simulink model "SingePhase_FB_Inverter_SPWM"  (R2023a)
settings: Solver=ode23t  StartTime=0.0  StopTime=0.1  MaxStep=1e-4  RelTol=1e-3
libraries: spsMosfetLib x8, spsSeriesRLCBranchLib x6, simulink x3, spsDCVoltageSourceLib x2, spsVoltageMeasurementLib x2, sps_lib x1
settings Model: Creator=Alielden  LastModifiedBy=Alielden
settings DataIOCC: SaveState=on  SignalLogging=off  DSMLogging=off  ReturnWorkspaceOutputs=off  LoggingToFile=on

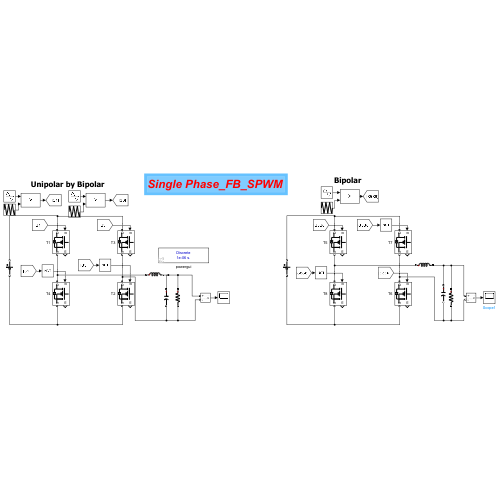
[thumbnail: Simulink's stored preview of the top-level diagram]
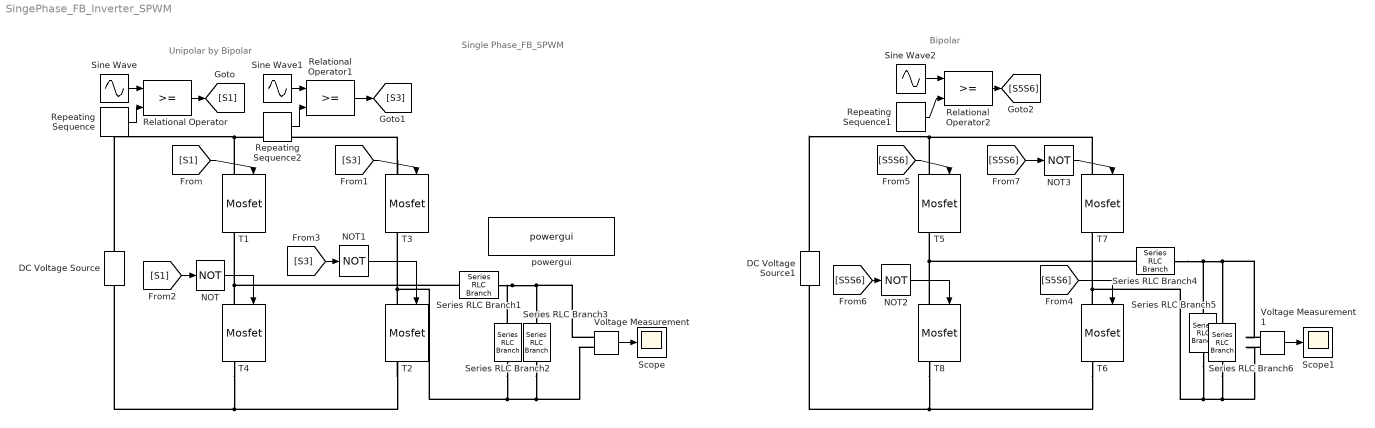
== system SingePhase_FB_Inverter_SPWM ==
  note: Unipolar by Bipolar
  note: Bipolar
  note: Single Phase_FB_SPWM
  DC Voltage Source : spsDCVoltageSourceLib/DC Voltage Source  Amplitude=100  Measurements=None
  DC Voltage Source1 : spsDCVoltageSourceLib/DC Voltage Source  Amplitude=100  Measurements=None
  NOT{,1..3} (4 alike) : Logic  Operator=NOT  AllPortsSameDT=off  OutDataTypeStr=boolean
  Relational Operator : RelationalOperator  OutDataTypeStr=boolean  RndMeth=Simplest  InputSameDT=off
  Relational Operator1 : RelationalOperator  OutDataTypeStr=boolean  RndMeth=Simplest  InputSameDT=off
  Relational Operator2 : RelationalOperator  OutDataTypeStr=boolean  RndMeth=Simplest  InputSameDT=off
  Repeating Sequence : simulink/Sources/Repeating Sequence  rep_seq_t=[0 (1/5000)/4 (1/5000)/2 (3/5000)/4 (1/5000)]  rep_seq_y=[0 1 0 -1 0]
  Repeating Sequence1 : simulink/Sources/Repeating Sequence  rep_seq_t=[0 (1/5000)/4 (1/5000)/2 (3/5000)/4 (1/5000)]  rep_seq_y=[0 1 0 -1 0]
  Repeating Sequence2 : simulink/Sources/Repeating Sequence  rep_seq_t=[0 (1/5000)/4 (1/5000)/2 (3/5000)/4 (1/5000)]  rep_seq_y=[0 1 0 -1 0]
  Scope : Scope
  Scope1 : Scope
  Series RLC Branch1 : spsSeriesRLCBranchLib/Series RLC Branch  LConnTagsString=__new0  RConnTagsString=__new0  BranchType=L  Resistance=10  Inductance=1e-3  SetiL0=off  InitialCurrent=0  Capacitance=1e-6  Setx0=off  InitialVoltage=0  Measurements=None
  Series RLC Branch2 : spsSeriesRLCBranchLib/Series RLC Branch  LConnTagsString=__new0  RConnTagsString=__new0  BranchType=C  Resistance=10  Inductance=1e-3  SetiL0=off  InitialCurrent=0  Capacitance=100e-6  Setx0=off  InitialVoltage=0  Measurements=None
  Series RLC Branch3 : spsSeriesRLCBranchLib/Series RLC Branch  LConnTagsString=__new0  RConnTagsString=__new0  BranchType=R  Resistance=10  Inductance=1e-3  SetiL0=off  InitialCurrent=0  Capacitance=1e-6  Setx0=off  InitialVoltage=0  Measurements=None
  Series RLC Branch4 : spsSeriesRLCBranchLib/Series RLC Branch  LConnTagsString=__new0  RConnTagsString=__new0  BranchType=L  Resistance=10  Inductance=1e-3  SetiL0=off  InitialCurrent=0  Capacitance=1e-6  Setx0=off  InitialVoltage=0  Measurements=None
  Series RLC Branch5 : spsSeriesRLCBranchLib/Series RLC Branch  LConnTagsString=__new0  RConnTagsString=__new0  BranchType=C  Resistance=10  Inductance=1e-3  SetiL0=off  InitialCurrent=0  Capacitance=100e-6  Setx0=off  InitialVoltage=0  Measurements=None
  Series RLC Branch6 : spsSeriesRLCBranchLib/Series RLC Branch  LConnTagsString=__new0  RConnTagsString=__new0  BranchType=R  Resistance=10  Inductance=1e-3  SetiL0=off  InitialCurrent=0  Capacitance=1e-6  Setx0=off  InitialVoltage=0  Measurements=None
  Sine Wave : Sin  Amplitude=.9  Frequency=2*pi*50  SampleTime=0
  Sine Wave1 : Sin  Amplitude=.9  Frequency=2*pi*50  Phase=180*pi/180  SampleTime=0
  Sine Wave2 : Sin  Amplitude=.9  Frequency=2*pi*50  SampleTime=0
  T{1..8} (8 alike) : spsMosfetLib/Mosfet  Ron=0.1  Lon=0  Rd=0.01  Vfd=0  IC=0  Rs=1e5  Cs=inf  Measurements=on
  Voltage Measurement : spsVoltageMeasurementLib/Voltage Measurement  PhasorSimulation=off  OutputType=Complex  PSBequivalent=0
  Voltage Measurement1 : spsVoltageMeasurementLib/Voltage Measurement  PhasorSimulation=off  OutputType=Complex  PSBequivalent=0
  powergui : sps_lib/powergui  Priority=1  SimulationMode=Discrete  SampleTime=1e-6  frequency=60  Iterations=50  frequencyindice=0  Pbase=100e6  ErrMax=1e-4  UnitsV=kV  UnitsW=MW  buscounter=0  FunctionMessages=off  echomessages=off  EnableUseOfTLC=off  CurrentSourceSwitches=off  DisableSnubberDevices=off  DisableRonSwitches=off  DisableVfSwitches=off  DisplayEquations=off  AutomaticDiscreteSolvers=off  SolverType=Tustin/Backward Euler (TBE)  Interpol=off  ExternalGateDelay=off  methode=off  Ts=100  x0status=blocks  SPID=on  SwTol=0  HookPort=off  NonlinearTolerance=1e-4  nMaxIteration=100  ContinueOnMaxIteration=off  RestoreLinks=warning  ResistiveCurrentMeasurement=off  Frange=[0:2:500]  Ylog=off  Xlog=on  ShowGrid=off  save=off  variable=ZData  structure=0  ZoomFFT=off  StartTime=0.0  cycles=1  DisplayStyle=1  fundamental=60  FreqAxis=off  MaxFrequency=1000  frequencyindicesteady=1  RmsSteady=1  display=off
  wires:
  Voltage Measurement/1 -> Scope/1
  NOT/1 -> T4/1
  NOT1/1 -> T2/1
  Sine Wave/1 -> Relational Operator/1
  Repeating Sequence/1 -> Relational Operator/2
  Sine Wave1/1 -> Relational Operator1/1
  Repeating Sequence2/1 -> Relational Operator1/2
  Voltage Measurement1/1 -> Scope1/1
  Sine Wave2/1 -> Relational Operator2/1
  Repeating Sequence1/1 -> Relational Operator2/2
  NOT2/1 -> T8/1
  NOT3/1 -> T7/1
  Relational Operator/1 -> [S1]
  Relational Operator1/1 -> [S3]
  [S1] -> T1/1
  [S3] -> T3/1
  [S1] -> NOT/1
  [S3] -> NOT1/1
  Relational Operator2/1 -> [S5S6]
  [S5S6] -> T6/1
  [S5S6] -> T5/1
  [S5S6] -> NOT2/1
  [S5S6] -> NOT3/1
  connections:
  T2/LConn1 -- T3/RConn1 -- Series RLC Branch3/RConn1 -- Voltage Measurement/LConn2 -- Series RLC Branch2/RConn1
  T3/LConn1 -- DC Voltage Source/RConn1 -- T1/LConn1
  T2/RConn1 -- T4/RConn1 -- DC Voltage Source/LConn1
  T4/LConn1 -- T1/RConn1 -- Series RLC Branch1/LConn1
  Series RLC Branch1/RConn1 -- Series RLC Branch3/LConn1 -- Voltage Measurement/LConn1 -- Series RLC Branch2/LConn1
  T6/LConn1 -- Voltage Measurement1/LConn2 -- Series RLC Branch6/RConn1 -- Series RLC Branch5/RConn1 -- T7/RConn1
  DC Voltage Source1/LConn1 -- T6/RConn1 -- T8/RConn1
  T5/LConn1 -- DC Voltage Source1/RConn1 -- T7/LConn1
  Series RLC Branch4/LConn1 -- T8/LConn1 -- T5/RConn1
  Series RLC Branch4/RConn1 -- Voltage Measurement1/LConn1 -- Series RLC Branch6/LConn1 -- Series RLC Branch5/LConn1
